simulink model "udpTestCoords"  (R2019b)
settings: Solver=FixedStepDiscrete  StartTime=0.0  StopTime=Inf  FixedStep=1/30  RelTol=1e-3
InitFcn:
  | tb = twinbeam('147.32.86.177', 30000);
  | tb.coords_subs(30006);
  | 
  | pause(1)
StopFcn:
  | tb.coords_unsubs();
  | 
  | delete(tb);
model workspace (MAT data in the model file):
  NumberOfBeads = Simulink.Parameter
  NumberOfBeads.Value = 1
  NumberOfBeads.DataType = 'auto'
  NumberOfBeads.Dimensions = [1 1]
undefined symbols (not defined in the file or in its folder): f
libraries: instrumentlib x1, simulink x1
settings Model: EnablePacing=on  ParameterArgumentNames=NumberOfBeads  OrderedModelArguments=off  Creator=marti  LastModifiedBy=gurtnmar
settings RTWCC: Description=Generic Real-Time Target  RTWCompilerOptimization=on
settings CodeAppCC: MaxIdLength=95

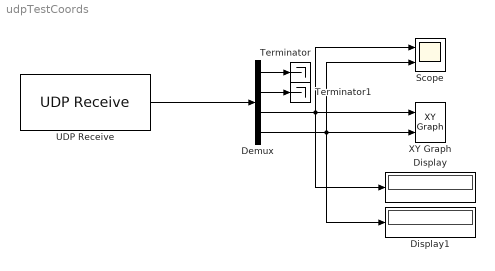
== system udpTestCoords ==
  Demux : Demux
  Display : Display
  Display1 : Display
  Scope : Scope  NumInputPorts=2
  Terminator : Terminator
  Terminator1 : Terminator
  UDP Receive : instrumentlib/UDP Receive  Host=147.32.86.177  Port=57504  LocalPort=30006  EnablePortSharing=off  GetLatestData=on  DataSize="[4  1]"  DataType=uint16  ASCIIFormatting=%f,  Terminator=LF  ByteOrder=LittleEndian  EnableBlockingMode=on  Timeout=4  SampleTime=-1  LocalAddress=147.32.86.128
  XY Graph : simulink/Sinks/XY Graph  xmin=-1  xmax=1  ymin=-1  ymax=1  st=-1
  wires:
  UDP Receive/1 -> Demux/1
  Demux/1 -> Terminator/1
  Demux/2 -> Terminator1/1
  Demux/3 -> Display/1, Scope/1, XY Graph/1
  Demux/4 -> Display1/1, Scope/2, XY Graph/2
